simulink model "sgMdl_IO751_IO752_PROFINETLoopback"  (R2024b)
settings: Solver=FixedStepAuto  StartTime=0.0  StopTime=inf  RelTol=1e-3  EnableMultiTasking=on
undefined symbols (not defined in the file): C, Ts
libraries: slrealtimeutilitieslib x54, speedgoatlib_IO751 x3, speedgoatlib_IO752 x3, simulink x2
Description:
  | IO751 & IO752 - PROFINET Loopback
settings Model: ModifiedByFormat=Speedgoat  Creator=Speedgoat  LastModifiedBy=Speedgoat
settings SolverCC: ConcurrentTasks=on  AlgebraicLoopSolver=TrustRegion  PositivePriorityOrder=on  AutoInsertRateTranBlk=on  InsertRTBMode=Never (minimum delay)
settings DataIOCC: SaveFormat=Array  SaveState=on  SignalLoggingName=logsOut
settings OptimizationCC: BlockReduction=off  BooleanDataType=off  OptimizeBlockIOStorage=off  BufferReuse=off  ReuseModelBlockBuffer=off  GlobalBufferReuse=off  ExpressionFolding=off  LocalBlockOutputs=off  InitFltsAndDblsToZero=on  OptimizeDataStoreBuffers=off  BusAssignmentInplaceUpdate=off
settings DebuggingCC: SaveWithParameterizedLinksMsg=none  UnderspecifiedInitializationDetection=Classic  MergeDetectMultiDrivingBlocksExec=none  CheckExecutionContextPreStartOutputMsg=on  SignalResolutionControl=TryResolveAllWithWarning  TasksWithSamePriorityMsg=none  UnconnectedInputMsg=warning  UnconnectedOutputMsg=warning  UnconnectedLineMsg=warning  SFUnexpectedBacktrackingDiag=warning  SFNoUnconditionalDefaultTransitionDiag=warning  SFExecutionAtInitializationDiag=none  ArithmeticOperatorsInVariantConditions=warning
settings HardwareCC: ProdBitPerLong=64  ProdLongLongMode=on  ProdHWDeviceType=Intel->x86-64 (Linux 64)
settings ModelReferenceCC: EnableRefExpFcnMdlSchedulingChecks=on  PropagateSignalLabelsOutOfModel=off
settings SFSimCC: SimUseLocalCustomCode=off  SimTargetLang=C++
settings RTWCC: Description=Speedgoat Real-Time Target Machine  SystemTargetFile=speedgoat.tlc  TemplateMakefile=slrealtime_default_tmf  RTWUseLocalCustomCode=off  Toolchain=Simulink Real-Time Toolchain  BuildConfiguration=Faster Runs  TargetLang=C++  GPUComputeCapability=3.5  DLArmComputeVersion=19.05
settings CodeAppCC: StateflowObjectComments=on
settings SimulinkRealTimeTargetCC: SubcomponentCodeInterfacePackaging=Reusable function  InstructionSetFMA=off  LogToMDFFile=off  SLRTFileLogMaxRuns=10
settings ConfigComp: CovMetricSettings=dw  CovSaveCumulativeToWorkspaceVar=on  CovSaveSingleToWorkspaceVar=on  CovExternalEMLEnable=off  CovSFcnEnable=off  CovBoundaryAbsTol=1.0e-5

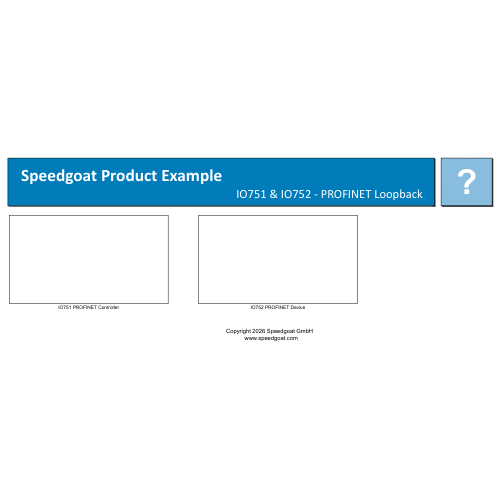
[thumbnail: Simulink's stored preview of the top-level diagram]
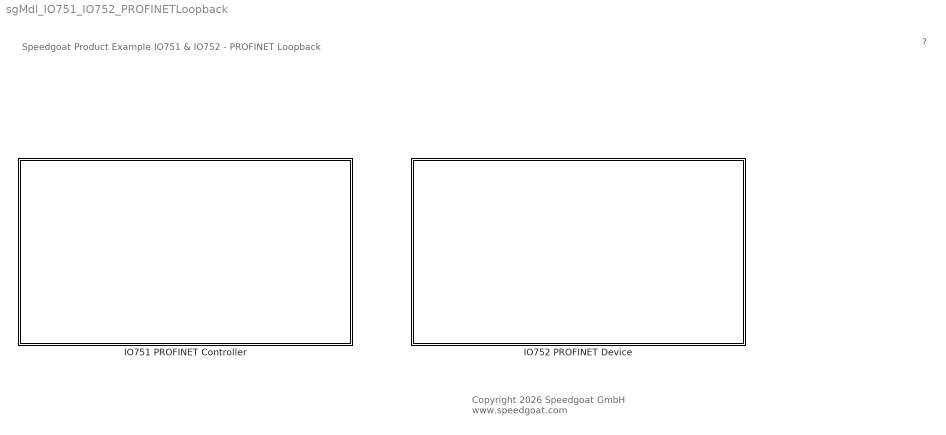
== system sgMdl_IO751_IO752_PROFINETLoopback ==
  note: Speedgoat Product Example
      | IO751 & IO752 - PROFINET Loopback
  note: ?
  note: Copyright 2026 Speedgoat GmbH
      |  www.speedgoat.com
  IO751 PROFINET Controller : Subsystem
  IO752 PROFINET Device : Subsystem

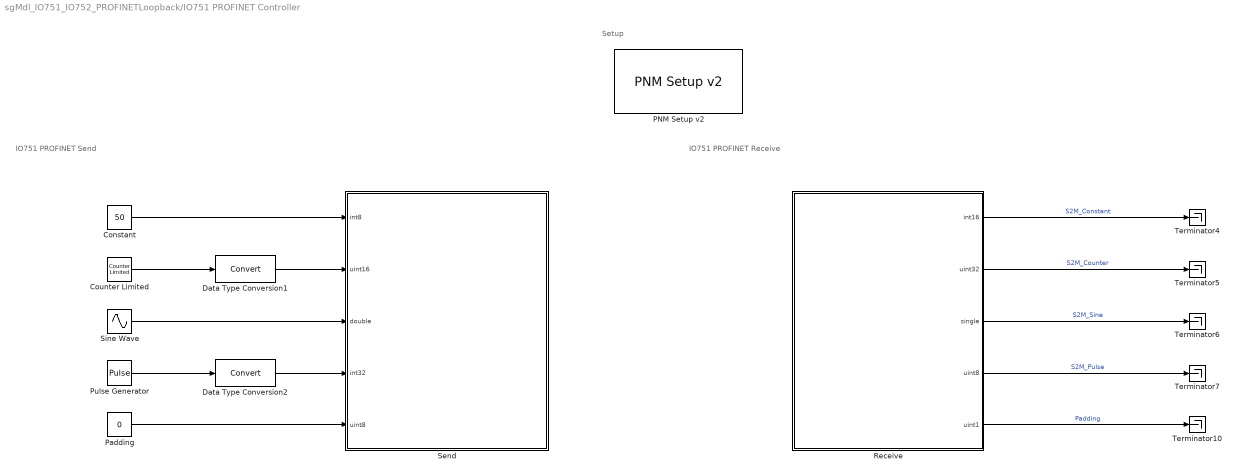
== system sgMdl_IO751_IO752_PROFINETLoopback/IO751 PROFINET Controller ==
  note: IO751 PROFINET Receive
  note: IO751 PROFINET Send
  note: Setup
  Constant : Constant  Value=50  OutDataTypeStr=Inherit: Inherit via back propagation  SampleTime=Ts
  Counter Limited : simulink/Sources/Counter Limited  uplimit=100  tsamp=Ts/Ts/10
  Data Type Conversion1 : DataTypeConversion  SaturateOnIntegerOverflow=off  RndMeth=Floor
  Data Type Conversion2 : DataTypeConversion  SaturateOnIntegerOverflow=off  RndMeth=Floor
  "PNM Setup v2 " : speedgoatlib_IO751/PNM Setup v2   id=1  driveLetter=C:  configurationMode=Configuration file  mode=Polling mode  pciSlot=-1  quantityOfAcyclicObjects=0  qtyMods=[1,0,0]  ConfigFile=which('IO751_IO752_Loopback_m.nxd')  parOptAcyclic=off  protocol=IO751  firmware=PROFINET Controller
      settings: SourceProductName=IO751 PROFINET Controller
  Padding : Constant  Value=0  OutDataTypeStr=Inherit: Inherit via back propagation  SampleTime=Ts
  Pulse Generator : DiscretePulseGenerator  Amplitude=100  Period=2*1/Ts  PulseWidth=1/Ts  SampleTime=Ts
  Receive : Subsystem
  Send : Subsystem
  Sine Wave : Sin  Amplitude=100  Frequency=2*pi  Phase=pi  SampleTime=Ts
  Terminator{4..7,10} (5 alike) : Terminator
  wires:
  Sine Wave/1 -> Send/3(double)
  Counter Limited/1 -> Data Type Conversion1/1
  Constant/1 -> Send/1(int8)
  Receive/1(int16) -> Terminator4/1  "S2M_Constant"
  Receive/2(uint32) -> Terminator5/1  "S2M_Counter"
  Receive/3(single) -> Terminator6/1  "S2M_Sine"
  Receive/4(uint8) -> Terminator7/1  "S2M_Pulse"
  Data Type Conversion1/1 -> Send/2(uint16)
  Data Type Conversion2/1 -> Send/4(int32)
  Padding/1 -> Send/5(uint8)
  Pulse Generator/1 -> Data Type Conversion2/1
  Receive/5(uint1) -> Terminator10/1  "Padding"

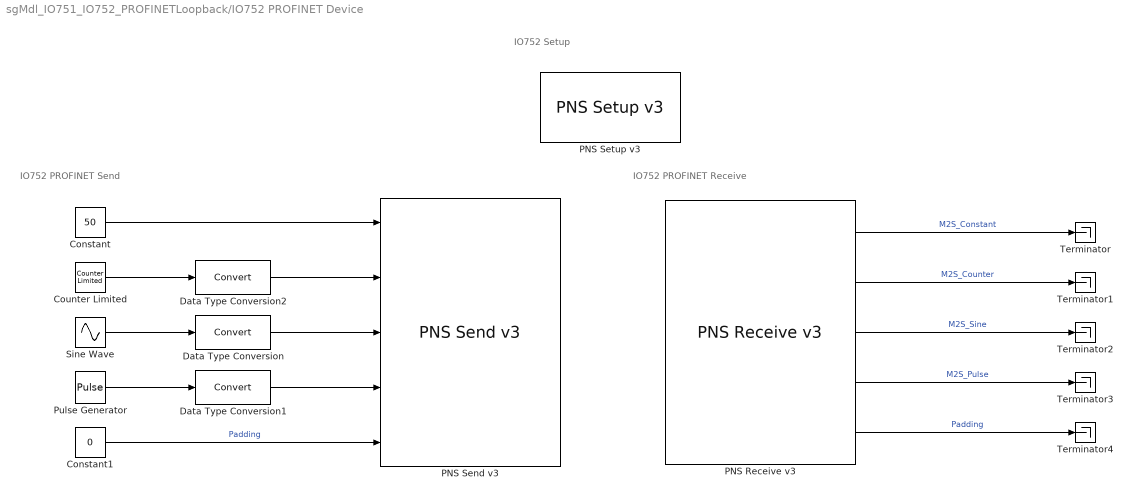
== system sgMdl_IO751_IO752_PROFINETLoopback/IO752 PROFINET Device ==
  note: IO752 Setup
  note: IO752 PROFINET Send
  note: IO752 PROFINET Receive
  Constant : Constant  Value=50  OutDataTypeStr=Inherit: Inherit via back propagation  SampleTime=Ts
  Constant1 : Constant  Value=0  OutDataTypeStr=uint8
  Counter Limited : simulink/Sources/Counter Limited  uplimit=100  tsamp=Ts/Ts/10
  Data Type Conversion : DataTypeConversion  SaturateOnIntegerOverflow=off  RndMeth=Floor
  Data Type Conversion1 : DataTypeConversion  SaturateOnIntegerOverflow=off  RndMeth=Floor
  Data Type Conversion2 : DataTypeConversion  SaturateOnIntegerOverflow=off  RndMeth=Floor
  PNS Receive v3 : speedgoatlib_IO752/PNS Receive v3  id=2  SampleTime=Ts  DataLevel=Data Item  GroupDataItems=off  PortLabel1=off  PortLabel2=on  PortLabel3=off  PnModuleConfig="{ '0', '', 'SG IO752 V4.8.0.0', '12625', '', '', 'DAP V4.8.0.0', '0', '', '', '1', ''; '0', '1', '  SG IO752 V4.8.0.0', '12625', '12624', '', 'DAP V4.8.0.0', '1', '', '', '', ''; '0', '32768', '  PN-IO', '12625', '12625', '', 'Interfacesubmodule', '1', '', '', '', ''; '0', '32769', '  Port 1', '12625', '12370', '', 'Port1Submodule', '1', '', '', '', ''; '0', '32770', '  Port 2', '12625', '12370', '', 'Port2Submodule', '1', '', '', '', ''; '1', '', 'Int16 Input', '12', '', '', 'int16input', '0', '', '', '', ''; '1', '1', '  Int16 Input', '12', '13', '', 'int16input', '1', '{\"int16\",[4],[1]}', '', '', ''; '2', '', 'Uint32 Input', '6', '', '', 'uint32input', '0', '', '', '', ''; '2', '1', '  Uint32 Input', '6', '7', '', 'uint32input', '1', '{\"uint32\",[7],[1]}', '', '', ''; '3', '', 'Single Input', '4', '', '', 'singleinput', '0', '', '', '', ''; '3', '1', '  Single Input', '4', '5', '', 'singleinput', '1', '{\"single\",[1],[1]}', '', '', ''; '4', '', 'Uint8 Input', '14', '', '', 'uint8input', '0', '', '', '', ''; '4', '1', '  Uint8 Input', '14', '15', '', 'uint8input', '1', '{\"uint8\",[3],[1]}', '', '', ''; '5', '', 'Uint8 Input', '14', '', '', 'uint8input', '0', '', '', '', ''; '5', '1', '  Uint8 Input', '14', '15', '', 'uint8input', '1', '{\"uint8\",[3],[1]}', '', '', ''; '6', '', 'Int8 Output', '46', '', '', 'int8output', '0', '', '', '', ''; '6', '1', '  Int8 Output', '46', '47', '', 'int8output', '1', '', '{\"int8\",[2],[1]}', '', ''; '7', '', 'Uint16 Output', '40', '', '', 'uint16output', '0', '', '', '', ''; '7', '1', '  Uint16 Output', '40', '41', '', 'uint16output', '1', '', '{\"uint16\",[5],[1]}', '', ''; '8', '', 'Double Output', '32', '', '', 'doubleoutput', '0', '', '', '', ''; '8', '1', '  Double Output', '32', '33', '', 'doubleoutput', '1', '', '{\"double\",[0],[1]}', '', ''; '9', '', 'Int32 Output', '38', '', '', 'int32output', '0', '', '', '', ''; '9', '1', '  Int32 Output', '38', '39', '', 'int32output', '1', '', '{\"int32\",[6],[1]}', '', ''; '10', '', 'Uint8 Output', '44', '', '', 'uint8output', '0', '', '', '', ''; '10', '1', '  Uint8 Output', '44', '45', '', 'uint8output', '1', '', '{\"uint8\",[3],[1]}', '', '' }"
      settings: SourceProductName=IO752 PROFINET Device
  PNS Send v3 : speedgoatlib_IO752/PNS Send v3  id=2  SampleTime=Ts  DataLevel=Data Item  GroupDataItems=off  PortLabel1=off  PortLabel2=on  PortLabel3=off  PnModuleConfig="{ '0', '', 'SG IO752 V4.8.0.0', '12625', '', '', 'DAP V4.8.0.0', '0', '', '', '1', ''; '0', '1', '  SG IO752 V4.8.0.0', '12625', '12624', '', 'DAP V4.8.0.0', '1', '', '', '', ''; '0', '32768', '  PN-IO', '12625', '12625', '', 'Interfacesubmodule', '1', '', '', '', ''; '0', '32769', '  Port 1', '12625', '12370', '', 'Port1Submodule', '1', '', '', '', ''; '0', '32770', '  Port 2', '12625', '12370', '', 'Port2Submodule', '1', '', '', '', ''; '1', '', 'Int16 Input', '12', '', '', 'int16input', '0', '', '', '', ''; '1', '1', '  Int16 Input', '12', '13', '', 'int16input', '1', '{\"int16\",[4],[1]}', '', '', ''; '2', '', 'Uint32 Input', '6', '', '', 'uint32input', '0', '', '', '', ''; '2', '1', '  Uint32 Input', '6', '7', '', 'uint32input', '1', '{\"uint32\",[7],[1]}', '', '', ''; '3', '', 'Single Input', '4', '', '', 'singleinput', '0', '', '', '', ''; '3', '1', '  Single Input', '4', '5', '', 'singleinput', '1', '{\"single\",[1],[1]}', '', '', ''; '4', '', 'Uint8 Input', '14', '', '', 'uint8input', '0', '', '', '', ''; '4', '1', '  Uint8 Input', '14', '15', '', 'uint8input', '1', '{\"uint8\",[3],[1]}', '', '', ''; '5', '', 'Uint8 Input', '14', '', '', 'uint8input', '0', '', '', '', ''; '5', '1', '  Uint8 Input', '14', '15', '', 'uint8input', '1', '{\"uint8\",[3],[1]}', '', '', ''; '6', '', 'Int8 Output', '46', '', '', 'int8output', '0', '', '', '', ''; '6', '1', '  Int8 Output', '46', '47', '', 'int8output', '1', '', '{\"int8\",[2],[1]}', '', ''; '7', '', 'Uint16 Output', '40', '', '', 'uint16output', '0', '', '', '', ''; '7', '1', '  Uint16 Output', '40', '41', '', 'uint16output', '1', '', '{\"uint16\",[5],[1]}', '', ''; '8', '', 'Double Output', '32', '', '', 'doubleoutput', '0', '', '', '', ''; '8', '1', '  Double Output', '32', '33', '', 'doubleoutput', '1', '', '{\"double\",[0],[1]}', '', ''; '9', '', 'Int32 Output', '38', '', '', 'int32output', '0', '', '', '', ''; '9', '1', '  Int32 Output', '38', '39', '', 'int32output', '1', '', '{\"int32\",[6],[1]}', '', ''; '10', '', 'Uint8 Output', '44', '', '', 'uint8output', '0', '', '', '', ''; '10', '1', '  Uint8 Output', '44', '45', '', 'uint8output', '1', '', '{\"uint8\",[3],[1]}', '', '' }"
      settings: SourceProductName=IO752 PROFINET Device
  PNS Setup v3 : speedgoatlib_IO752/PNS Setup v3  id=2  PciSlot=-1  StationName='sgiopns'  BusStart=On model start  SystemRedundancy=off  RecordSuccess=on  GsdFile=[speedgoatroot, '\sg_blocks\cifx\eds\GSDML-V2.43-Speedgoat-IO752-20241009.xml']  VendorId=1985  DeviceId=1  OptionalIdentity=off  DeviceType='sgiopns'  OrderId='2X752'  HwRev=1  SwRevPrefix='V'  SwRev=[4,8,0]  SerialNumber='0'  ModuleConfigTable="{ '0', '', 'SG IO752 V4.8.0.0', '12625', '', '', 'DAP V4.8.0.0', '0', '', '', '1', ''; '0', '1', '  SG IO752 V4.8.0.0', '12625', '12624', '', 'DAP V4.8.0.0', '1', '', '', '', ''; '0', '32768', '  PN-IO', '12625', '12625', '', 'Interfacesubmodule', '1', '', '', '', ''; '0', '32769', '  Port 1', '12625', '12370', '', 'Port1Submodule', '1', '', '', '', ''; '0', '32770', '  Port 2', '12625', '12370', '', 'Port2Submodule', '1', '', '', '', ''; '1', '', 'Int16 Input', '12', '', '', 'int16input', '0', '', '', '', ''; '1', '1', '  Int16 Input', '12', '13', '', 'int16input', '1', '{\"int16\",[4],[1]}', '', '', ''; '2', '', 'Uint32 Input', '6', '', '', 'uint32input', '0', '', '', '', ''; '2', '1', '  Uint32 Input', '6', '7', '', 'uint32input', '1', '{\"uint32\",[7],[1]}', '', '', ''; '3', '', 'Single Input', '4', '', '', 'singleinput', '0', '', '', '', ''; '3', '1', '  Single Input', '4', '5', '', 'singleinput', '1', '{\"single\",[1],[1]}', '', '', ''; '4', '', 'Uint8 Input', '14', '', '', 'uint8input', '0', '', '', '', ''; '4', '1', '  Uint8 Input', '14', '15', '', 'uint8input', '1', '{\"uint8\",[3],[1]}', '', '', ''; '5', '', 'Uint8 Input', '14', '', '', 'uint8input', '0', '', '', '', ''; '5', '1', '  Uint8 Input', '14', '15', '', 'uint8input', '1', '{\"uint8\",[3],[1]}', '', '', ''; '6', '', 'Int8 Output', '46', '', '', 'int8output', '0', '', '', '', ''; '6', '1', '  Int8 Output', '46', '47', '', 'int8output', '1', '', '{\"int8\",[2],[1]}', '', ''; '7', '', 'Uint16 Output', '40', '', '', 'uint16output', '0', '', '', '', ''; '7', '1', '  Uint16 Output', '40', '41', '', 'uint16output', '1', '', '{\"uint16\",[5],[1]}', '', ''; '8', '', 'Double Output', '32', '', '', 'doubleoutput', '0', '', '', '', ''; '8', '1', '  Double Output', '32', '33', '', 'doubleoutput', '1', '', '{\"double\",[0],[1]}', '', ''; '9', '', 'Int32 Output', '38', '', '', 'int32output', '0', '', '', '', ''; '9', '1', '  Int32 Output', '38', '39', '', 'int32output', '1', '', '{\"int32\",[6],[1]}', '', ''; '10', '', 'Uint8 Output', '44', '', '', 'uint8output', '0', '', '', '', ''; '10', '1', '  Uint8 Output', '44', '45', '', 'uint8output', '1', '', '{\"uint8\",[3],[1]}', '', '' }"
      settings: SourceProductName=IO752 PROFINET Device
  Pulse Generator : DiscretePulseGenerator  Amplitude=100  Period=2*1/Ts  PulseWidth=1/Ts  SampleTime=Ts
  Sine Wave : Sin  Amplitude=100  Frequency=2*pi  Phase=pi  SampleTime=Ts
  Terminator{,1..4} (5 alike) : Terminator
  wires:
  PNS Receive v3/2 -> Terminator1/1  "M2S_Counter"
  PNS Receive v3/3 -> Terminator2/1  "M2S_Sine"
  PNS Receive v3/4 -> Terminator3/1  "M2S_Pulse"
  Constant/1 -> PNS Send v3/1
  Counter Limited/1 -> Data Type Conversion2/1
  Sine Wave/1 -> Data Type Conversion/1
  Data Type Conversion/1 -> PNS Send v3/3
  Data Type Conversion1/1 -> PNS Send v3/4
  Data Type Conversion2/1 -> PNS Send v3/2
  Pulse Generator/1 -> Data Type Conversion1/1
  Constant1/1 -> PNS Send v3/5  "Padding"
  PNS Receive v3/5 -> Terminator4/1  "Padding"
  PNS Receive v3/1 -> Terminator/1  "M2S_Constant"

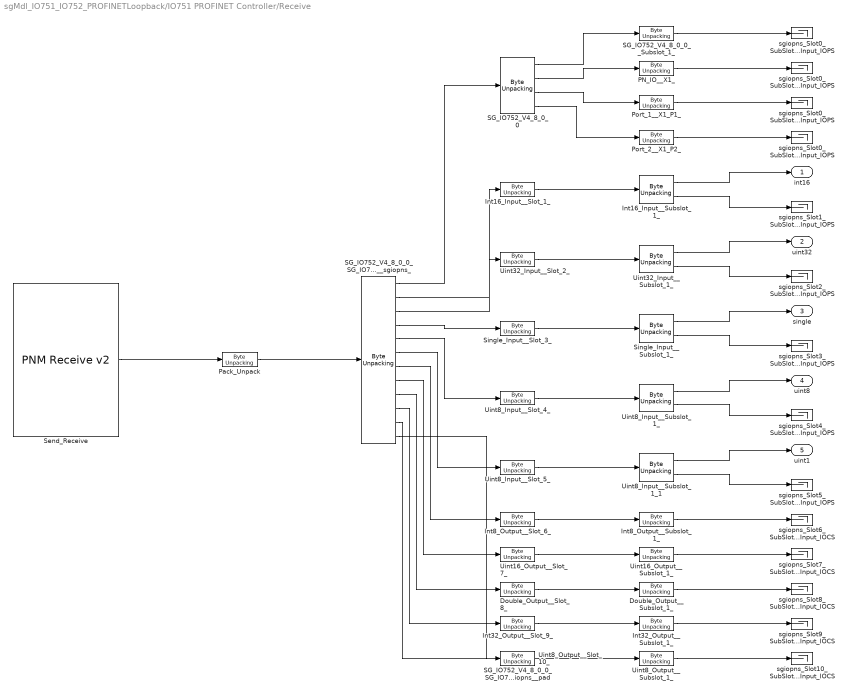
== system sgMdl_IO751_IO752_PROFINETLoopback/IO751 PROFINET Controller/Receive ==
  Double_Output__Slot_8_ : slrealtimeutilitieslib/Byte Unpacking  MaskUnpackedDataTypes={'uint8'}  MaskUnpackedDataSizes={[1]}  MaskAlignment=1
  Double_Output__Subslot_1_ : slrealtimeutilitieslib/Byte Unpacking  MaskUnpackedDataTypes={'uint8'}  MaskUnpackedDataSizes={[1]}  MaskAlignment=1
  Int16_Input__Slot_1_ : slrealtimeutilitieslib/Byte Unpacking  MaskUnpackedDataTypes={'uint8'}  MaskUnpackedDataSizes={[3]}  MaskAlignment=1
  Int16_Input__Subslot_1_ : slrealtimeutilitieslib/Byte Unpacking  MaskUnpackedDataTypes={'int16','uint8'}  MaskUnpackedDataSizes={[1],[1]}  MaskAlignment=1
  Int32_Output__Slot_9_ : slrealtimeutilitieslib/Byte Unpacking  MaskUnpackedDataTypes={'uint8'}  MaskUnpackedDataSizes={[1]}  MaskAlignment=1
  Int32_Output__Subslot_1_ : slrealtimeutilitieslib/Byte Unpacking  MaskUnpackedDataTypes={'uint8'}  MaskUnpackedDataSizes={[1]}  MaskAlignment=1
  Int8_Output__Slot_6_ : slrealtimeutilitieslib/Byte Unpacking  MaskUnpackedDataTypes={'uint8'}  MaskUnpackedDataSizes={[1]}  MaskAlignment=1
  Int8_Output__Subslot_1_ : slrealtimeutilitieslib/Byte Unpacking  MaskUnpackedDataTypes={'uint8'}  MaskUnpackedDataSizes={[1]}  MaskAlignment=1
  PN_IO__X1_ : slrealtimeutilitieslib/Byte Unpacking  MaskUnpackedDataTypes={'uint8'}  MaskUnpackedDataSizes={[1]}  MaskAlignment=1
  Pack_Unpack : slrealtimeutilitieslib/Byte Unpacking  MaskUnpackedDataTypes={'uint8'}  MaskUnpackedDataSizes={[28]}  MaskAlignment=1
  Port_1__X1_P1_ : slrealtimeutilitieslib/Byte Unpacking  MaskUnpackedDataTypes={'uint8'}  MaskUnpackedDataSizes={[1]}  MaskAlignment=1
  Port_2__X1_P2_ : slrealtimeutilitieslib/Byte Unpacking  MaskUnpackedDataTypes={'uint8'}  MaskUnpackedDataSizes={[1]}  MaskAlignment=1
  SG_IO752_V4_8_0_0 : slrealtimeutilitieslib/Byte Unpacking  MaskUnpackedDataTypes={'uint8','uint8','uint8','uint8'}  MaskUnpackedDataSizes={[1],[1],[1],[1]}  MaskAlignment=1
  SG_IO752_V4_8_0_0_SG_IO752_V4_8_0_0__sgiopns_ : slrealtimeutilitieslib/Byte Unpacking  MaskUnpackedDataTypes={'uint8','uint8','uint8','uint8','uint8','uint8','uint8','uint8','uint8','uint8','uint8','uint8'}  MaskUnpackedDataSizes={[4],[3],[5],[5],[2],[2],[1],[1],[1],[1],[1],[2]}  MaskAlignment=1
  SG_IO752_V4_8_0_0_SG_IO752_V4_8_0_0__sgiopns__pad : Terminator
  SG_IO752_V4_8_0_0__Subslot_1_ : slrealtimeutilitieslib/Byte Unpacking  MaskUnpackedDataTypes={'uint8'}  MaskUnpackedDataSizes={[1]}  MaskAlignment=1
  Send_Receive : speedgoatlib_IO751/PNM Receive v2   id=1  portType=1 port with n element vector of type UINT8  inputOutput=28  sampleTime=-1
      settings: SourceProductName=IO751 PROFINET Controller
  Single_Input__Slot_3_ : slrealtimeutilitieslib/Byte Unpacking  MaskUnpackedDataTypes={'uint8'}  MaskUnpackedDataSizes={[5]}  MaskAlignment=1
  Single_Input__Subslot_1_ : slrealtimeutilitieslib/Byte Unpacking  MaskUnpackedDataTypes={'single','uint8'}  MaskUnpackedDataSizes={[1],[1]}  MaskAlignment=1
  Uint16_Output__Slot_7_ : slrealtimeutilitieslib/Byte Unpacking  MaskUnpackedDataTypes={'uint8'}  MaskUnpackedDataSizes={[1]}  MaskAlignment=1
  Uint16_Output__Subslot_1_ : slrealtimeutilitieslib/Byte Unpacking  MaskUnpackedDataTypes={'uint8'}  MaskUnpackedDataSizes={[1]}  MaskAlignment=1
  Uint32_Input__Slot_2_ : slrealtimeutilitieslib/Byte Unpacking  MaskUnpackedDataTypes={'uint8'}  MaskUnpackedDataSizes={[5]}  MaskAlignment=1
  Uint32_Input__Subslot_1_ : slrealtimeutilitieslib/Byte Unpacking  MaskUnpackedDataTypes={'uint32','uint8'}  MaskUnpackedDataSizes={[1],[1]}  MaskAlignment=1
  Uint8_Input__Slot_4_ : slrealtimeutilitieslib/Byte Unpacking  MaskUnpackedDataTypes={'uint8'}  MaskUnpackedDataSizes={[2]}  MaskAlignment=1
  Uint8_Input__Slot_5_ : slrealtimeutilitieslib/Byte Unpacking  MaskUnpackedDataTypes={'uint8'}  MaskUnpackedDataSizes={[2]}  MaskAlignment=1
  Uint8_Input__Subslot_1_ : slrealtimeutilitieslib/Byte Unpacking  MaskUnpackedDataTypes={'uint8','uint8'}  MaskUnpackedDataSizes={[1],[1]}  MaskAlignment=1
  Uint8_Input__Subslot_1_1 : slrealtimeutilitieslib/Byte Unpacking  MaskUnpackedDataTypes={'uint8','uint8'}  MaskUnpackedDataSizes={[1],[1]}  MaskAlignment=1
  Uint8_Output__Slot_10_ : slrealtimeutilitieslib/Byte Unpacking  MaskUnpackedDataTypes={'uint8'}  MaskUnpackedDataSizes={[1]}  MaskAlignment=1
  Uint8_Output__Subslot_1_ : slrealtimeutilitieslib/Byte Unpacking  MaskUnpackedDataTypes={'uint8'}  MaskUnpackedDataSizes={[1]}  MaskAlignment=1
  sgiopns_Slot0_SubSlot1_Input_IOPS : Terminator
  sgiopns_Slot0_SubSlot32768_Input_IOPS : Terminator
  sgiopns_Slot0_SubSlot32769_Input_IOPS : Terminator
  sgiopns_Slot0_SubSlot32770_Input_IOPS : Terminator
  sgiopns_Slot10_SubSlot1_Input_IOCS : Terminator
  sgiopns_Slot1_SubSlot1_Input_IOPS : Terminator
  sgiopns_Slot2_SubSlot1_Input_IOPS : Terminator
  sgiopns_Slot3_SubSlot1_Input_IOPS : Terminator
  sgiopns_Slot4_SubSlot1_Input_IOPS : Terminator
  sgiopns_Slot5_SubSlot1_Input_IOPS : Terminator
  sgiopns_Slot6_SubSlot1_Input_IOCS : Terminator
  sgiopns_Slot7_SubSlot1_Input_IOCS : Terminator
  sgiopns_Slot8_SubSlot1_Input_IOCS : Terminator
  sgiopns_Slot9_SubSlot1_Input_IOCS : Terminator
  int16 : Outport  OutDataTypeStr=int16  PortDimensions=1
  uint32 : Outport  Port=2  OutDataTypeStr=uint32  PortDimensions=1
  single : Outport  Port=3  OutDataTypeStr=single  PortDimensions=1
  uint8 : Outport  Port=4  OutDataTypeStr=uint8  PortDimensions=1
  uint1 : Outport  Port=5  OutDataTypeStr=uint8  PortDimensions=1
  wires:
  SG_IO752_V4_8_0_0__Subslot_1_/1 -> sgiopns_Slot0_SubSlot1_Input_IOPS/1
  PN_IO__X1_/1 -> sgiopns_Slot0_SubSlot32768_Input_IOPS/1
  Port_1__X1_P1_/1 -> sgiopns_Slot0_SubSlot32769_Input_IOPS/1
  Port_2__X1_P2_/1 -> sgiopns_Slot0_SubSlot32770_Input_IOPS/1
  SG_IO752_V4_8_0_0/1 -> SG_IO752_V4_8_0_0__Subslot_1_/1
  SG_IO752_V4_8_0_0/2 -> PN_IO__X1_/1
  SG_IO752_V4_8_0_0/3 -> Port_1__X1_P1_/1
  SG_IO752_V4_8_0_0/4 -> Port_2__X1_P2_/1
  Int16_Input__Subslot_1_/1 -> int16/1
  Int16_Input__Subslot_1_/2 -> sgiopns_Slot1_SubSlot1_Input_IOPS/1
  Int16_Input__Slot_1_/1 -> Int16_Input__Subslot_1_/1
  Uint32_Input__Subslot_1_/1 -> uint32/1
  Uint32_Input__Subslot_1_/2 -> sgiopns_Slot2_SubSlot1_Input_IOPS/1
  Uint32_Input__Slot_2_/1 -> Uint32_Input__Subslot_1_/1
  Single_Input__Subslot_1_/1 -> single/1
  Single_Input__Subslot_1_/2 -> sgiopns_Slot3_SubSlot1_Input_IOPS/1
  Single_Input__Slot_3_/1 -> Single_Input__Subslot_1_/1
  Uint8_Input__Subslot_1_/1 -> uint8/1
  Uint8_Input__Subslot_1_/2 -> sgiopns_Slot4_SubSlot1_Input_IOPS/1
  Uint8_Input__Slot_4_/1 -> Uint8_Input__Subslot_1_/1
  Uint8_Input__Subslot_1_1/1 -> uint1/1
  Uint8_Input__Subslot_1_1/2 -> sgiopns_Slot5_SubSlot1_Input_IOPS/1
  Uint8_Input__Slot_5_/1 -> Uint8_Input__Subslot_1_1/1
  Int8_Output__Subslot_1_/1 -> sgiopns_Slot6_SubSlot1_Input_IOCS/1
  Int8_Output__Slot_6_/1 -> Int8_Output__Subslot_1_/1
  Uint16_Output__Subslot_1_/1 -> sgiopns_Slot7_SubSlot1_Input_IOCS/1
  Uint16_Output__Slot_7_/1 -> Uint16_Output__Subslot_1_/1
  Double_Output__Subslot_1_/1 -> sgiopns_Slot8_SubSlot1_Input_IOCS/1
  Double_Output__Slot_8_/1 -> Double_Output__Subslot_1_/1
  Int32_Output__Subslot_1_/1 -> sgiopns_Slot9_SubSlot1_Input_IOCS/1
  Int32_Output__Slot_9_/1 -> Int32_Output__Subslot_1_/1
  Uint8_Output__Subslot_1_/1 -> sgiopns_Slot10_SubSlot1_Input_IOCS/1
  Uint8_Output__Slot_10_/1 -> Uint8_Output__Subslot_1_/1
  SG_IO752_V4_8_0_0_SG_IO752_V4_8_0_0__sgiopns_/1 -> SG_IO752_V4_8_0_0/1
  SG_IO752_V4_8_0_0_SG_IO752_V4_8_0_0__sgiopns_/2 -> Int16_Input__Slot_1_/1
  SG_IO752_V4_8_0_0_SG_IO752_V4_8_0_0__sgiopns_/3 -> Uint32_Input__Slot_2_/1
  SG_IO752_V4_8_0_0_SG_IO752_V4_8_0_0__sgiopns_/4 -> Single_Input__Slot_3_/1
  SG_IO752_V4_8_0_0_SG_IO752_V4_8_0_0__sgiopns_/5 -> Uint8_Input__Slot_4_/1
  SG_IO752_V4_8_0_0_SG_IO752_V4_8_0_0__sgiopns_/6 -> Uint8_Input__Slot_5_/1
  SG_IO752_V4_8_0_0_SG_IO752_V4_8_0_0__sgiopns_/7 -> Int8_Output__Slot_6_/1
  SG_IO752_V4_8_0_0_SG_IO752_V4_8_0_0__sgiopns_/8 -> Uint16_Output__Slot_7_/1
  SG_IO752_V4_8_0_0_SG_IO752_V4_8_0_0__sgiopns_/9 -> Double_Output__Slot_8_/1
  SG_IO752_V4_8_0_0_SG_IO752_V4_8_0_0__sgiopns_/10 -> Int32_Output__Slot_9_/1
  SG_IO752_V4_8_0_0_SG_IO752_V4_8_0_0__sgiopns_/11 -> Uint8_Output__Slot_10_/1
  SG_IO752_V4_8_0_0_SG_IO752_V4_8_0_0__sgiopns_/12 -> SG_IO752_V4_8_0_0_SG_IO752_V4_8_0_0__sgiopns__pad/1
  Pack_Unpack/1 -> SG_IO752_V4_8_0_0_SG_IO752_V4_8_0_0__sgiopns_/1
  Send_Receive/1 -> Pack_Unpack/1

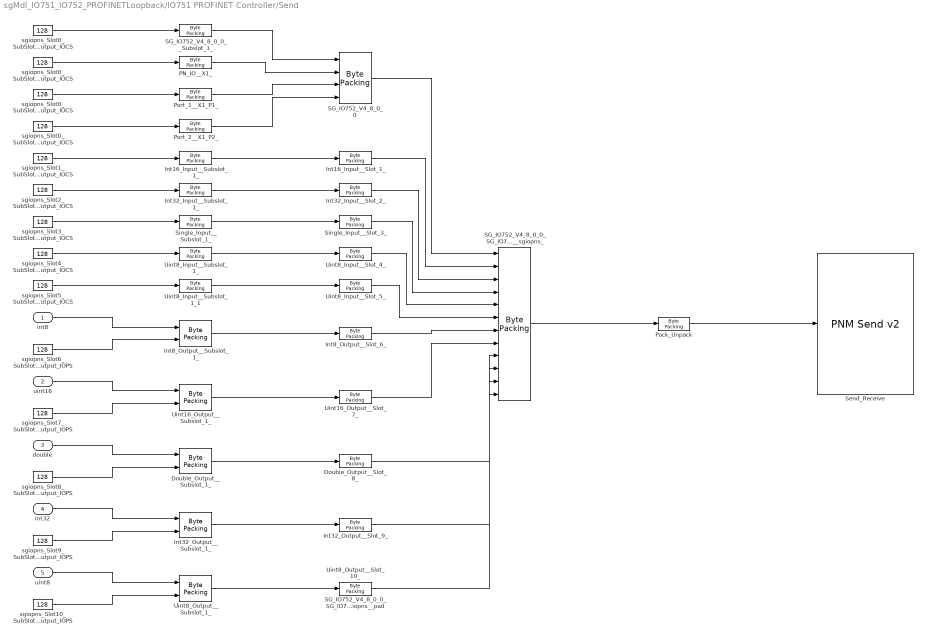
== system sgMdl_IO751_IO752_PROFINETLoopback/IO751 PROFINET Controller/Send ==
  int8 : Inport  OutDataTypeStr=int8  PortDimensions=1
  uint16 : Inport  Port=2  OutDataTypeStr=uint16  PortDimensions=1
  double : Inport  Port=3  OutDataTypeStr=double  PortDimensions=1
  int32 : Inport  Port=4  OutDataTypeStr=int32  PortDimensions=1
  uint8 : Inport  Port=5  OutDataTypeStr=uint8  PortDimensions=1
  Double_Output__Slot_8_ : slrealtimeutilitieslib/Byte Packing  MaskPackedDataType=uint8  MaskUnpackedDataTypes={'uint8'}  MaskAlignment=1
  Double_Output__Subslot_1_ : slrealtimeutilitieslib/Byte Packing  MaskPackedDataType=uint8  MaskUnpackedDataTypes={'double','uint8'}  MaskAlignment=1
  Int16_Input__Slot_1_ : slrealtimeutilitieslib/Byte Packing  MaskPackedDataType=uint8  MaskUnpackedDataTypes={'uint8'}  MaskAlignment=1
  Int16_Input__Subslot_1_ : slrealtimeutilitieslib/Byte Packing  MaskPackedDataType=uint8  MaskUnpackedDataTypes={'uint8'}  MaskAlignment=1
  Int32_Input__Slot_2_ : slrealtimeutilitieslib/Byte Packing  MaskPackedDataType=uint8  MaskUnpackedDataTypes={'uint8'}  MaskAlignment=1
  Int32_Input__Subslot_1_ : slrealtimeutilitieslib/Byte Packing  MaskPackedDataType=uint8  MaskUnpackedDataTypes={'uint8'}  MaskAlignment=1
  Int32_Output__Slot_9_ : slrealtimeutilitieslib/Byte Packing  MaskPackedDataType=uint8  MaskUnpackedDataTypes={'uint8'}  MaskAlignment=1
  Int32_Output__Subslot_1_ : slrealtimeutilitieslib/Byte Packing  MaskPackedDataType=uint8  MaskUnpackedDataTypes={'int32','uint8'}  MaskAlignment=1
  Int8_Output__Slot_6_ : slrealtimeutilitieslib/Byte Packing  MaskPackedDataType=uint8  MaskUnpackedDataTypes={'uint8'}  MaskAlignment=1
  Int8_Output__Subslot_1_ : slrealtimeutilitieslib/Byte Packing  MaskPackedDataType=uint8  MaskUnpackedDataTypes={'int8','uint8'}  MaskAlignment=1
  PN_IO__X1_ : slrealtimeutilitieslib/Byte Packing  MaskPackedDataType=uint8  MaskUnpackedDataTypes={'uint8'}  MaskAlignment=1
  Pack_Unpack : slrealtimeutilitieslib/Byte Packing  MaskPackedDataType=uint8  MaskUnpackedDataTypes={'uint8'}  MaskAlignment=1
  Port_1__X1_P1_ : slrealtimeutilitieslib/Byte Packing  MaskPackedDataType=uint8  MaskUnpackedDataTypes={'uint8'}  MaskAlignment=1
  Port_2__X1_P2_ : slrealtimeutilitieslib/Byte Packing  MaskPackedDataType=uint8  MaskUnpackedDataTypes={'uint8'}  MaskAlignment=1
  SG_IO752_V4_8_0_0 : slrealtimeutilitieslib/Byte Packing  MaskPackedDataType=uint8  MaskUnpackedDataTypes={'uint8','uint8','uint8','uint8'}  MaskAlignment=1
  SG_IO752_V4_8_0_0_SG_IO752_V4_8_0_0__sgiopns_ : slrealtimeutilitieslib/Byte Packing  MaskPackedDataType=uint8  MaskUnpackedDataTypes={'uint8','uint8','uint8','uint8','uint8','uint8','uint8','uint8','uint8','uint8','uint8','uint8'}  MaskAlignment=1
  SG_IO752_V4_8_0_0_SG_IO752_V4_8_0_0__sgiopns__pad : Constant  Value=[0 0]  OutDataTypeStr=uint8
  SG_IO752_V4_8_0_0__Subslot_1_ : slrealtimeutilitieslib/Byte Packing  MaskPackedDataType=uint8  MaskUnpackedDataTypes={'uint8'}  MaskAlignment=1
  Send_Receive : speedgoatlib_IO751/PNM Send v2   id=1  portType=1 port with n element vector of type UINT8  inputOutput=32  sampleTime=-1
      settings: SourceProductName=IO751 PROFINET Controller
  Single_Input__Slot_3_ : slrealtimeutilitieslib/Byte Packing  MaskPackedDataType=uint8  MaskUnpackedDataTypes={'uint8'}  MaskAlignment=1
  Single_Input__Subslot_1_ : slrealtimeutilitieslib/Byte Packing  MaskPackedDataType=uint8  MaskUnpackedDataTypes={'uint8'}  MaskAlignment=1
  Uint16_Output__Slot_7_ : slrealtimeutilitieslib/Byte Packing  MaskPackedDataType=uint8  MaskUnpackedDataTypes={'uint8'}  MaskAlignment=1
  Uint16_Output__Subslot_1_ : slrealtimeutilitieslib/Byte Packing  MaskPackedDataType=uint8  MaskUnpackedDataTypes={'uint16','uint8'}  MaskAlignment=1
  Uint8_Input__Slot_4_ : slrealtimeutilitieslib/Byte Packing  MaskPackedDataType=uint8  MaskUnpackedDataTypes={'uint8'}  MaskAlignment=1
  Uint8_Input__Slot_5_ : slrealtimeutilitieslib/Byte Packing  MaskPackedDataType=uint8  MaskUnpackedDataTypes={'uint8'}  MaskAlignment=1
  Uint8_Input__Subslot_1_ : slrealtimeutilitieslib/Byte Packing  MaskPackedDataType=uint8  MaskUnpackedDataTypes={'uint8'}  MaskAlignment=1
  Uint8_Input__Subslot_1_1 : slrealtimeutilitieslib/Byte Packing  MaskPackedDataType=uint8  MaskUnpackedDataTypes={'uint8'}  MaskAlignment=1
  Uint8_Output__Slot_10_ : slrealtimeutilitieslib/Byte Packing  MaskPackedDataType=uint8  MaskUnpackedDataTypes={'uint8'}  MaskAlignment=1
  Uint8_Output__Subslot_1_ : slrealtimeutilitieslib/Byte Packing  MaskPackedDataType=uint8  MaskUnpackedDataTypes={'uint8','uint8'}  MaskAlignment=1
  sgiopns_Slot0_SubSlot1_Output_IOCS : Constant  Value=128  OutDataTypeStr=uint8
  sgiopns_Slot0_SubSlot32768_Output_IOCS : Constant  Value=128  OutDataTypeStr=uint8
  sgiopns_Slot0_SubSlot32769_Output_IOCS : Constant  Value=128  OutDataTypeStr=uint8
  sgiopns_Slot0_SubSlot32770_Output_IOCS : Constant  Value=128  OutDataTypeStr=uint8
  sgiopns_Slot10_SubSlot1_Output_IOPS : Constant  Value=128  OutDataTypeStr=uint8
  sgiopns_Slot1_SubSlot1_Output_IOCS : Constant  Value=128  OutDataTypeStr=uint8
  sgiopns_Slot2_SubSlot1_Output_IOCS : Constant  Value=128  OutDataTypeStr=uint8
  sgiopns_Slot3_SubSlot1_Output_IOCS : Constant  Value=128  OutDataTypeStr=uint8
  sgiopns_Slot4_SubSlot1_Output_IOCS : Constant  Value=128  OutDataTypeStr=uint8
  sgiopns_Slot5_SubSlot1_Output_IOCS : Constant  Value=128  OutDataTypeStr=uint8
  sgiopns_Slot6_SubSlot1_Output_IOPS : Constant  Value=128  OutDataTypeStr=uint8
  sgiopns_Slot7_SubSlot1_Output_IOPS : Constant  Value=128  OutDataTypeStr=uint8
  sgiopns_Slot8_SubSlot1_Output_IOPS : Constant  Value=128  OutDataTypeStr=uint8
  sgiopns_Slot9_SubSlot1_Output_IOPS : Constant  Value=128  OutDataTypeStr=uint8
  wires:
  sgiopns_Slot0_SubSlot1_Output_IOCS/1 -> SG_IO752_V4_8_0_0__Subslot_1_/1
  sgiopns_Slot0_SubSlot32768_Output_IOCS/1 -> PN_IO__X1_/1
  sgiopns_Slot0_SubSlot32769_Output_IOCS/1 -> Port_1__X1_P1_/1
  sgiopns_Slot0_SubSlot32770_Output_IOCS/1 -> Port_2__X1_P2_/1
  SG_IO752_V4_8_0_0__Subslot_1_/1 -> SG_IO752_V4_8_0_0/1
  PN_IO__X1_/1 -> SG_IO752_V4_8_0_0/2
  Port_1__X1_P1_/1 -> SG_IO752_V4_8_0_0/3
  Port_2__X1_P2_/1 -> SG_IO752_V4_8_0_0/4
  sgiopns_Slot1_SubSlot1_Output_IOCS/1 -> Int16_Input__Subslot_1_/1
  Int16_Input__Subslot_1_/1 -> Int16_Input__Slot_1_/1
  sgiopns_Slot2_SubSlot1_Output_IOCS/1 -> Int32_Input__Subslot_1_/1
  Int32_Input__Subslot_1_/1 -> Int32_Input__Slot_2_/1
  sgiopns_Slot3_SubSlot1_Output_IOCS/1 -> Single_Input__Subslot_1_/1
  Single_Input__Subslot_1_/1 -> Single_Input__Slot_3_/1
  sgiopns_Slot4_SubSlot1_Output_IOCS/1 -> Uint8_Input__Subslot_1_/1
  Uint8_Input__Subslot_1_/1 -> Uint8_Input__Slot_4_/1
  sgiopns_Slot5_SubSlot1_Output_IOCS/1 -> Uint8_Input__Subslot_1_1/1
  Uint8_Input__Subslot_1_1/1 -> Uint8_Input__Slot_5_/1
  int8/1 -> Int8_Output__Subslot_1_/1
  sgiopns_Slot6_SubSlot1_Output_IOPS/1 -> Int8_Output__Subslot_1_/2
  Int8_Output__Subslot_1_/1 -> Int8_Output__Slot_6_/1
  uint16/1 -> Uint16_Output__Subslot_1_/1
  sgiopns_Slot7_SubSlot1_Output_IOPS/1 -> Uint16_Output__Subslot_1_/2
  Uint16_Output__Subslot_1_/1 -> Uint16_Output__Slot_7_/1
  double/1 -> Double_Output__Subslot_1_/1
  sgiopns_Slot8_SubSlot1_Output_IOPS/1 -> Double_Output__Subslot_1_/2
  Double_Output__Subslot_1_/1 -> Double_Output__Slot_8_/1
  int32/1 -> Int32_Output__Subslot_1_/1
  sgiopns_Slot9_SubSlot1_Output_IOPS/1 -> Int32_Output__Subslot_1_/2
  Int32_Output__Subslot_1_/1 -> Int32_Output__Slot_9_/1
  uint8/1 -> Uint8_Output__Subslot_1_/1
  sgiopns_Slot10_SubSlot1_Output_IOPS/1 -> Uint8_Output__Subslot_1_/2
  Uint8_Output__Subslot_1_/1 -> Uint8_Output__Slot_10_/1
  SG_IO752_V4_8_0_0/1 -> SG_IO752_V4_8_0_0_SG_IO752_V4_8_0_0__sgiopns_/1
  Int16_Input__Slot_1_/1 -> SG_IO752_V4_8_0_0_SG_IO752_V4_8_0_0__sgiopns_/2
  Int32_Input__Slot_2_/1 -> SG_IO752_V4_8_0_0_SG_IO752_V4_8_0_0__sgiopns_/3
  Single_Input__Slot_3_/1 -> SG_IO752_V4_8_0_0_SG_IO752_V4_8_0_0__sgiopns_/4
  Uint8_Input__Slot_4_/1 -> SG_IO752_V4_8_0_0_SG_IO752_V4_8_0_0__sgiopns_/5
  Uint8_Input__Slot_5_/1 -> SG_IO752_V4_8_0_0_SG_IO752_V4_8_0_0__sgiopns_/6
  Int8_Output__Slot_6_/1 -> SG_IO752_V4_8_0_0_SG_IO752_V4_8_0_0__sgiopns_/7
  Uint16_Output__Slot_7_/1 -> SG_IO752_V4_8_0_0_SG_IO752_V4_8_0_0__sgiopns_/8
  Double_Output__Slot_8_/1 -> SG_IO752_V4_8_0_0_SG_IO752_V4_8_0_0__sgiopns_/9
  Int32_Output__Slot_9_/1 -> SG_IO752_V4_8_0_0_SG_IO752_V4_8_0_0__sgiopns_/10
  Uint8_Output__Slot_10_/1 -> SG_IO752_V4_8_0_0_SG_IO752_V4_8_0_0__sgiopns_/11
  SG_IO752_V4_8_0_0_SG_IO752_V4_8_0_0__sgiopns__pad/1 -> SG_IO752_V4_8_0_0_SG_IO752_V4_8_0_0__sgiopns_/12
  SG_IO752_V4_8_0_0_SG_IO752_V4_8_0_0__sgiopns_/1 -> Pack_Unpack/1
  Pack_Unpack/1 -> Send_Receive/1
